simulink library "Feeder3_lib"  (Simulink 8.1)
settings: Solver=ode45  StartTime=0.0  StopTime=10.0  RelTol=1e-3
undefined symbols (not defined in the file): cable_spec, cb_mech_delay, Left, Ts, type, V
libraries: breaker_lib x11, transformer_lib x5, cables_lib x5, Load_lib x5, ssn_lib x3, rtlab x2, artemis x2
settings Model: Creator=re25624  LastModifiedBy=re25624

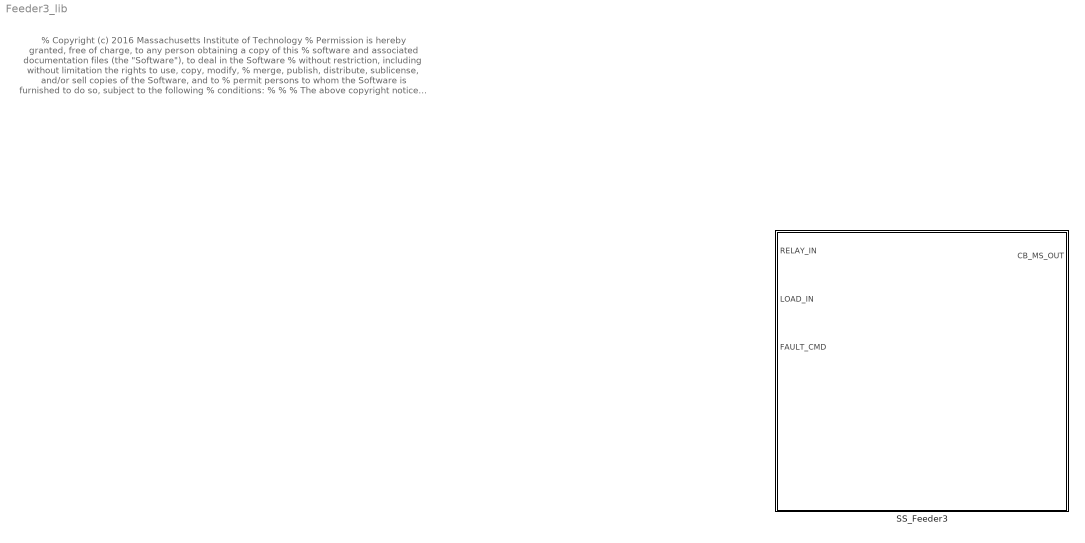
== system Feeder3_lib ==
  note: % Copyright (c) 2016 Massachusetts Institute of Technology
      | % Permission is hereby granted, free of charge, to any person obtaining a copy of this
      | % software and associated documentation files (the "Software"), to deal in the Software
      | % without restriction, including without limitation the rights to use, copy, modify,
      | % merge, publish, distribute, sublicense, and/or sell copies of the Software, and to
      | % permit persons to whom the Software is furnished to do so, subject to the following
      | % conditions:
      | %
      | %
      | % The above copyright notice and this permission notice shall be included in
      | % all copies or substantial portions of the Software.
      | %
      | % THE SOFTWARE IS PROVIDED "AS IS", WITHOUT WARRANTY OF ANY KIND, EXPRESS OR IMPLIED,
      | % INCLUDING BUT NOT LIMITED TO THE WARRANTIES OF MERCHANTABILITY, FITNESS FOR A
      | % PARTICULAR PURPOSE AND NONINFRINGEMENT. IN NO EVENT SHALL THE AUTHORS OR COPYRIGHT
      | % HOLDERS BE LIABLE FOR ANY CLAIM, DAMAGES OR OTHER LIABILITY, WHETHER IN AN ACTION
      | % OF CONTRACT, TORT OR OTHERWISE, ARISING FROM, OUT OF OR IN CONNECTION WITH THE
      | % SOFTWARE OR THE USE OR OTHER DEALINGS IN THE SOFTWARE.
      | %
      | %
      | %%
  SS_Feeder3 : Subsystem

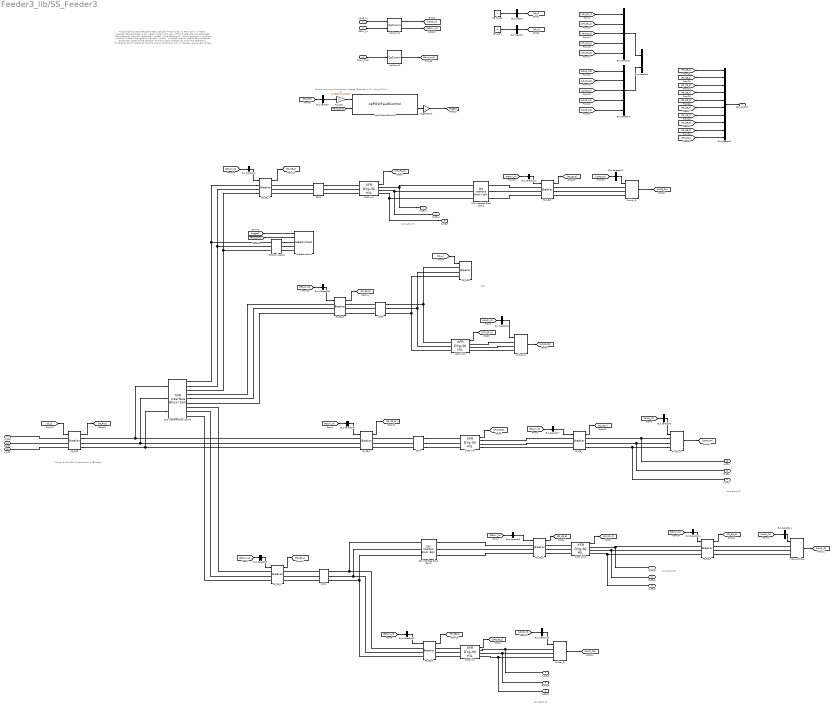
== system Feeder3_lib/SS_Feeder3 ==
  note: Point-on-wave synchronisation voltage (3-phase) in PU - Using 13.8 kV
  note: % Copyright (c) 2016 Massachusetts Institute of Technology
      | % Permission is hereby granted, free of charge, to any person obtaining a copy of this
      | % software and associated documentation files (the "Software"), to deal in the Software
      | % without restriction, including without limitation the rights to use, copy, modify,
      | % merge, publish, distribute, sublicense, and/or sell copies of the Software, and to
      | % permit persons to whom the Software is furnished to do so, subject to the following
      | % conditions:
      | %
      | %
      | % The above copyright notice and this permission notice shall be included in
      | % all copies or substantial portions of the Software.
      | %
      | % THE SOFTWARE IS PROVIDED "AS IS", WITHOUT WARRANTY OF ANY KIND, EXPRESS OR IMPLIED,
      | % INCLUDING BUT NOT LIMITED TO THE WARRANTIES OF MERCHANTABILITY, FITNESS FOR A
      | % PARTICULAR PURPOSE AND NONINFRINGEMENT. IN NO EVENT SHALL THE AUTHORS OR COPYRIGHT
      | % HOLDERS BE LIABLE FOR ANY CLAIM, DAMAGES OR OTHER LIABILITY, WHETHER IN AN ACTION
      | % OF CONTRACT, TORT OR OTHERWISE, ARISING FROM, OUT OF OR IN CONNECTION WITH THE
      | % SOFTWARE OR THE USE OR OTHER DEALINGS IN THE SOFTWARE.
      | %
      | %
      | %%
  note: connect to F1
  note: connect to F2
  note: connect to F2
  note: connect to F2
  note: CHP
  note: Signal for this Cb will come from a SEL relay
  RELAY_IN : Inport
  LOAD_IN : Inport  Port=2
  FAULT_CMD : Inport  Port=3
  1000 kVA : transformer_lib/XFR DYg-30 HIL  Rating=1000  Vp=13800  Vs=480  Z=5.56  XR=5.49
  1000 kVA1 : transformer_lib/XFR DYg-30 HIL  Rating=1000  Vp=13800  Vs=480  Z=5.56  XR=5.49
  2000 kVA : transformer_lib/XFR DYg-30 HIL  Rating=2000  Vp=13800  Vs=480  Z=5.75  XR=5.7
  2000 kVA1 : transformer_lib/XFR DYg-30 HIL  Rating=2000  Vp=13800  Vs=480  Z=5.75  XR=5.7
  2500 kVA : transformer_lib/XFR DYg-30 HIL  Rating=2500  Vp=13800  Vs=480  Z=5.75  XR=6.6
  500kcmil_cable : cables_lib/500kcmil_cable  length=1  par_sets=1
  Bus Creator : BusCreator  Inputs=1
  Bus Creator1 : BusCreator  Inputs=1
  Bus Creator2 : BusCreator  Inputs=5
  Bus Creator3 : BusCreator  Inputs=5
  Bus Creator4 : BusCreator  Inputs=2
  Bus Creator5 : BusCreator  Inputs=10
  Bus Selector : BusSelector  OutputSignals=Vabc_bus
  Bus Selector1 : BusSelector  OutputSignals=F3_CB_4
  Bus Selector10 : BusSelector  OutputSignals=F3_CB_5
  Bus Selector11 : BusSelector  OutputSignals=P6
  Bus Selector12 : BusSelector  OutputSignals=F3_CB_9
  Bus Selector13 : BusSelector  OutputSignals=F3_CB_3
  Bus Selector14 : BusSelector  OutputSignals=F3_CB_8
  Bus Selector2 : BusSelector  OutputSignals=C6
  Bus Selector3 : BusSelector  OutputSignals=P4
  Bus Selector4 : BusSelector  OutputSignals=I6
  Bus Selector5 : BusSelector  OutputSignals=C5
  Bus Selector6 : BusSelector  OutputSignals=F3_CB_2
  Bus Selector7 : BusSelector  OutputSignals=F3_CB_7
  Bus Selector8 : BusSelector  OutputSignals=F3_CB_6
  Bus Selector9 : BusSelector  OutputSignals=F3_CB_1
  C301 : cables_lib/PI-Section  cable_spec=[cable_spec(13, :)]  line_length=2500  parallel_sets=1
  C302 : cables_lib/PI-Section  cable_spec=[cable_spec(11, :)]  line_length=2000  parallel_sets=1
  C303 : cables_lib/PI-Section  cable_spec=[cable_spec(13, :)]  line_length=2000  parallel_sets=1
  C304 : cables_lib/PI-Section  cable_spec=[cable_spec(11, :)]  line_length=1500  parallel_sets=2
  CB closed : Constant
  CB open : Constant  Value=0
  Critical_5 : Load_lib/Dynamic_Load  V=460  Ts=Ts
  Critical_6 : Load_lib/Dynamic_Load  V=460  Ts=Ts
  F3_CB_{1..9} (9 alike) : breaker_lib/Breaker  Ts=Ts  mech_delays=[cb_mech_delay(1,:)]
  F3_GCB : breaker_lib/Breaker  Ts=Ts  mech_delays=[cb_mech_delay(1,:)]
  F3_PCC : breaker_lib/Breaker  Ts=Ts  mech_delays=[cb_mech_delay(1,:)]
  Interruptible_6 : Load_lib/Dynamic_Load  V=460  Ts=Ts
  OpComm1 : rtlab/OpComm  nbport=2  groupe_acq=1  subsys_rate=0  st=0  Synchronization=on  Interpolation=on  Threshold=1.0  Missed_Data=off  Sim_Time=off  Samples=off  dynSigOut=off  from_console=0  warning_done=off  writeOpCommFile=off  Offset=off
  OpComm2 : rtlab/OpComm  nbport=1  groupe_acq=1  subsys_rate=0  st=0  Synchronization=on  Interpolation=on  Threshold=1.0  Missed_Data=off  Sim_Time=off  Samples=off  dynSigOut=off  from_console=1  warning_done=off  writeOpCommFile=off  Offset=off
  Priority_4 : Load_lib/Dynamic_Load  V=460  Ts=Ts
  Priority_6 : Load_lib/Dynamic_Load  V=460  Ts=Ts
  SSN Interface Block (3ph)1 : ssn_lib/SSN Interface Block (3ph)  nb_phase=3  nb_port=2  p1_type=V-type(Left)  p2_type=V-type (Right)  p3_type=V-type(Left)  p4_type=V-type(Left)  p5_type=V-type(Left)  p6_type=V-type(Left)  p7_type=V-type(Left)  p8_type=V-type(Left)  p9_type=V-type(Left)  p10_type=V-type(Left)  p11_type=V-type(Left)  p12_type=V-type(Left)  p13_type=V-type(Left)  p14_type=V-type(Left)  p15_type=V-type(Left)  p16_type=V-type(Left)  I_port_shunt_resistance=1e9
  SSN Interface Block (3ph)2 : ssn_lib/SSN Interface Block (3ph)  nb_phase=3  nb_port=2  p1_type=V-type(Left)  p2_type=V-type (Right)  p3_type=V-type(Left)  p4_type=V-type(Left)  p5_type=V-type(Left)  p6_type=V-type(Left)  p7_type=V-type(Left)  p8_type=V-type(Left)  p9_type=V-type(Left)  p10_type=V-type(Left)  p11_type=V-type(Left)  p12_type=V-type(Left)  p13_type=V-type(Left)  p14_type=V-type(Left)  p15_type=V-type(Left)  p16_type=V-type(Left)  I_port_shunt_resistance=1e9
  SSN Interface Block (3ph)5 : ssn_lib/SSN Interface Block (3ph)  nb_phase=3  nb_port=4  p1_type=V-type(Left)  p2_type=V-type (Right)  p3_type=V-type (Right)  p4_type=V-type (Right)  p5_type=V-type(Left)  p6_type=V-type(Left)  p7_type=V-type(Left)  p8_type=V-type(Left)  p9_type=V-type(Left)  p10_type=V-type(Left)  p11_type=V-type(Left)  p12_type=V-type(Left)  p13_type=V-type(Left)  p14_type=V-type(Left)  p15_type=V-type(Left)  p16_type=V-type(Left)  I_port_shunt_resistance=1e9
  a : Gain  Gain=1/(13800*sqrt(2/3))
  opElectricFault : artemis/Tools /POW faults/opElectricFault  FaultLocation=location 4  FaultResistance=0.0001  GroundResistance=0.0001  InitialStates=[0 0 0]  SnubberResistance=1e6  SnubberCapacitance=inf
  opPOWFaultControl1 : artemis/Tools /POW faults/opPOWFaultControl  Ts=Ts  usePLL=off  Fgrid=60  PLL_k=[180 3200 1]  vol_sel=1: rising zero-corssing  SyncPhase_menu=A  T_acq=0.8
  triggerFAULT : Gain
  A_CB_4 : PMIOPort  Port=1  Side=Right
  B_CB_4 : PMIOPort  Port=2  Side=Right
  C_CB_4 : PMIOPort  Port=3  Side=Right
  A_CB_5 : PMIOPort  Port=4  Side=Right
  B_CB_5 : PMIOPort  Port=5  Side=Right
  C_CB_5 : PMIOPort  Port=6  Side=Right
  A_CB_6 : PMIOPort  Port=7  Side=Right
  B_CB_6 : PMIOPort  Port=8  Side=Right
  C_CB_6 : PMIOPort  Port=9  Side=Right
  A_CB_7 : PMIOPort  Port=10  Side=Right
  B_CB_7 : PMIOPort  Port=11  Side=Right
  C_CB_7 : PMIOPort  Port=12  Side=Right
  A_PCC : PMIOPort  Port=13  Side=Left
  B_PCC : PMIOPort  Port=14  Side=Left
  C_PCC : PMIOPort  Port=15  Side=Left
  CB_MS_OUT : Outport
  wires:
  FAULT_CMD/1 -> OpComm2/1
  OpComm2/1 -> [fault_cmd]
  [trigger] -> opElectricFault/1
  [fault_cmd] -> opElectricFault/2
  a/1 -> opPOWFaultControl1/1
  Bus Selector/1 -> a/1  "<Vabc_bus>"
  [F3_PCC] -> Bus Selector/1
  triggerFAULT/1 -> [trigger]  "triggerFAULTsig"
  opPOWFaultControl1/2 -> triggerFAULT/1
  [fault_cmd] -> opPOWFaultControl1/2
  [F3_CB_9] -> Bus Creator5/9  "F3_CB_9"
  [F3_CB_8] -> Bus Creator5/8  "F3_CB_8"
  [RELAY_IN] -> Bus Selector14/1
  Bus Selector14/1 -> F3_CB_8/1  "<F3_CB_8>"
  F3_CB_8/1 -> [F3_CB_8]
  [RELAY_IN] -> Bus Selector12/1
  Bus Selector12/1 -> F3_CB_9/1  "<F3_CB_9>"
  F3_CB_9/1 -> [F3_CB_9]
  [LOAD_P6] -> Bus Creator3/5  "F3_P6"
  Priority_6/1 -> [LOAD_P6]
  Bus Selector11/1 -> Priority_6/1  "<P6>"
  [LOAD_IN] -> Bus Selector11/1
  [F3_PCC] -> Bus Creator5/10  "F3_PCC"
  F3_PCC/1 -> [F3_PCC]
  F3_CB_7/1 -> [F3_CB_7]
  2500 kVA/1 -> [XFM_F3_5]
  [cb_o] -> F3_GCB/1
  [cb_c] -> F3_PCC/1
  [RELAY_IN] -> Bus Selector13/1
  Bus Selector13/1 -> F3_CB_3/1  "<F3_CB_3>"
  [RELAY_IN] -> Bus Selector10/1
  Bus Selector10/1 -> F3_CB_5/1  "<F3_CB_5>"
  [RELAY_IN] -> Bus Selector9/1
  Bus Selector9/1 -> F3_CB_1/1  "<F3_CB_1>"
  [RELAY_IN] -> Bus Selector8/1
  Bus Selector8/1 -> F3_CB_6/1  "<F3_CB_6>"
  [RELAY_IN] -> Bus Selector7/1
  Bus Selector7/1 -> F3_CB_7/1  "<F3_CB_7>"
  [RELAY_IN] -> Bus Selector6/1
  Bus Selector6/1 -> F3_CB_2/1  "<F3_CB_2>"
  OpComm1/2 -> [RELAY_IN]
  RELAY_IN/1 -> OpComm1/2
  [RELAY_IN] -> Bus Selector1/1
  Bus Creator5/1 -> CB_MS_OUT/1
  [F3_CB_4] -> Bus Creator5/4  "F3_CB_4"
  [F3_CB_2] -> Bus Creator5/2  "F3_CB_2"
  [F3_CB_3] -> Bus Creator5/3  "F3_CB_3"
  [F3_CB_6] -> Bus Creator5/6  "F3_CB_6"
  [F3_CB_7] -> Bus Creator5/7  "F3_CB_7"
  [F3_CB_5] -> Bus Creator5/5  "F3_CB_5"
  [F3_CB_1] -> Bus Creator5/1  "F3_CB_1"
  F3_CB_5/1 -> [F3_CB_5]
  F3_CB_1/1 -> [F3_CB_1]
  F3_CB_6/1 -> [F3_CB_6]
  F3_CB_2/1 -> [F3_CB_2]
  F3_CB_3/1 -> [F3_CB_3]
  F3_CB_4/1 -> [F3_CB_4]
  Bus Creator3/1 -> Bus Creator4/2  "LOAD"
  Bus Creator2/1 -> Bus Creator4/1  "XFR"
  [LOAD_P4] -> Bus Creator3/4  "F3_P4"
  [LOAD_I6] -> Bus Creator3/3  "F3_I6"
  [LOAD_C5] -> Bus Creator3/1  "F3_C5"
  [LOAD_C6] -> Bus Creator3/2  "F3_C6"
  Critical_5/1 -> [LOAD_C5]
  Interruptible_6/1 -> [LOAD_I6]
  Priority_4/1 -> [LOAD_P4]
  Critical_6/1 -> [LOAD_C6]
  [XFM_F3_4] -> Bus Creator2/4  "F3_X4"
  [XFM_F3_3] -> Bus Creator2/3  "F3_X3"
  [XFM_F3_5] -> Bus Creator2/5  "F3_X5"
  [XFM_F3_1] -> Bus Creator2/1  "F3_X1"
  [XFM_F3_2] -> Bus Creator2/2  "F3_X2"
  1000 kVA1/1 -> [XFM_F3_4]
  1000 kVA/1 -> [XFM_F3_3]
  2000 kVA1/1 -> [XFM_F3_2]
  2000 kVA/1 -> [XFM_F3_1]
  Bus Selector5/1 -> Critical_5/1  "<C5>"
  Bus Selector4/1 -> Interruptible_6/1  "<I6>"
  Bus Selector3/1 -> Priority_4/1  "<P4>"
  Bus Selector2/1 -> Critical_6/1  "<C6>"
  [LOAD_IN] -> Bus Selector5/1
  [LOAD_IN] -> Bus Selector4/1
  [LOAD_IN] -> Bus Selector3/1
  [LOAD_IN] -> Bus Selector2/1
  OpComm1/1 -> [LOAD_IN]
  LOAD_IN/1 -> OpComm1/1
  CB open/1 -> Bus Creator1/1  "Logic_trip"
  Bus Selector1/1 -> F3_CB_4/1  "<F3_CB_4>"
  Bus Creator1/1 -> [cb_o]
  Bus Creator/1 -> [cb_c]
  CB closed/1 -> Bus Creator/1  "Logic_trip"
  connections:
  SSN Interface Block (3ph)2/RConn1 -- F3_CB_9/LConn1
  SSN Interface Block (3ph)2/RConn3 -- F3_CB_9/LConn3
  SSN Interface Block (3ph)2/RConn2 -- F3_CB_9/LConn2
  500kcmil_cable/RConn1 -- opElectricFault/LConn1
  500kcmil_cable/RConn3 -- opElectricFault/LConn3
  500kcmil_cable/RConn2 -- opElectricFault/LConn2
  SSN Interface Block (3ph)5/LConn2 -- F3_CB_2/LConn2 -- F3_PCC/RConn2
  SSN Interface Block (3ph)5/LConn3 -- F3_CB_2/LConn3 -- F3_PCC/RConn3
  SSN Interface Block (3ph)5/LConn1 -- F3_CB_2/LConn1 -- F3_PCC/RConn1
  F3_PCC/LConn1 -- A_PCC/RConn1
  F3_PCC/LConn3 -- C_PCC/RConn1
  F3_PCC/LConn2 -- B_PCC/RConn1
  C303/RConn1 -- 2500 kVA/LConn1
  C303/RConn3 -- 2500 kVA/LConn3
  C303/RConn2 -- 2500 kVA/LConn2
  C303/LConn3 -- F3_CB_4/RConn3
  C303/LConn2 -- F3_CB_4/RConn2
  C303/LConn1 -- F3_CB_4/RConn1
  SSN Interface Block (3ph)1/RConn3 -- F3_CB_6/LConn3
  SSN Interface Block (3ph)1/RConn1 -- F3_CB_6/LConn1
  SSN Interface Block (3ph)1/RConn2 -- F3_CB_6/LConn2
  F3_CB_1/LConn3 -- SSN Interface Block (3ph)5/RConn9
  F3_CB_1/LConn2 -- SSN Interface Block (3ph)5/RConn8
  F3_CB_1/LConn1 -- SSN Interface Block (3ph)5/RConn7
  SSN Interface Block (3ph)5/RConn5 -- F3_CB_3/LConn2
  SSN Interface Block (3ph)5/RConn6 -- F3_CB_3/LConn3
  SSN Interface Block (3ph)5/RConn4 -- F3_CB_3/LConn1
  F3_CB_4/LConn2 -- 500kcmil_cable/LConn2 -- SSN Interface Block (3ph)5/RConn2
  F3_CB_4/LConn3 -- 500kcmil_cable/LConn3 -- SSN Interface Block (3ph)5/RConn3
  F3_CB_4/LConn1 -- 500kcmil_cable/LConn1 -- SSN Interface Block (3ph)5/RConn1
  F3_CB_8/RConn3 -- Interruptible_6/LConn3
  F3_CB_8/RConn2 -- Interruptible_6/LConn2
  F3_CB_8/RConn1 -- Interruptible_6/LConn1
  F3_CB_9/RConn3 -- Priority_6/LConn3
  F3_CB_9/RConn2 -- Priority_6/LConn2
  F3_CB_9/RConn1 -- Priority_6/LConn1
  1000 kVA/RConn1 -- F3_CB_7/LConn1
  1000 kVA/RConn2 -- F3_CB_7/LConn2
  1000 kVA/RConn3 -- F3_CB_7/LConn3
  C304/RConn1 -- 1000 kVA/LConn1
  C304/RConn3 -- 1000 kVA/LConn3
  C304/RConn2 -- 1000 kVA/LConn2
  B_CB_4/RConn1 -- SSN Interface Block (3ph)2/LConn2 -- 2500 kVA/RConn2
  C_CB_4/RConn1 -- SSN Interface Block (3ph)2/LConn3 -- 2500 kVA/RConn3
  A_CB_4/RConn1 -- SSN Interface Block (3ph)2/LConn1 -- 2500 kVA/RConn1
  Critical_5/LConn2 -- B_CB_5/RConn1 -- 2000 kVA/RConn2
  Critical_5/LConn3 -- C_CB_5/RConn1 -- 2000 kVA/RConn3
  2000 kVA/RConn1 -- A_CB_5/RConn1 -- Critical_5/LConn1
  2000 kVA1/RConn2 -- B_CB_6/RConn1 -- F3_CB_8/LConn2
  F3_CB_8/LConn3 -- C_CB_6/RConn1 -- 2000 kVA1/RConn3
  2000 kVA1/RConn1 -- A_CB_6/RConn1 -- F3_CB_8/LConn1
  Priority_4/LConn2 -- B_CB_7/RConn1 -- F3_CB_7/RConn2
  Priority_4/LConn3 -- C_CB_7/RConn1 -- F3_CB_7/RConn3
  Priority_4/LConn1 -- A_CB_7/RConn1 -- F3_CB_7/RConn1
  C304/LConn3 -- F3_CB_2/RConn3
  F3_CB_5/RConn3 -- 2000 kVA/LConn3
  F3_CB_5/RConn1 -- 2000 kVA/LConn1
  C302/LConn1 -- F3_CB_3/RConn1
  F3_CB_6/RConn1 -- 2000 kVA1/LConn1
  C304/LConn2 -- F3_CB_2/RConn2
  SSN Interface Block (3ph)1/LConn2 -- C301/RConn2 -- F3_CB_5/LConn2
  C302/LConn3 -- F3_CB_3/RConn3
  F3_CB_5/RConn2 -- 2000 kVA/LConn2
  C301/LConn1 -- F3_CB_1/RConn1
  F3_GCB/LConn2 -- C302/RConn2 -- 1000 kVA1/LConn2
  F3_CB_6/RConn2 -- 2000 kVA1/LConn2
  F3_GCB/LConn1 -- C302/RConn1 -- 1000 kVA1/LConn1
  C302/LConn2 -- F3_CB_3/RConn2
  F3_GCB/LConn3 -- C302/RConn3 -- 1000 kVA1/LConn3
  C304/LConn1 -- F3_CB_2/RConn1
  C301/LConn3 -- F3_CB_1/RConn3
  Critical_6/LConn3 -- 1000 kVA1/RConn3
  SSN Interface Block (3ph)1/LConn3 -- C301/RConn3 -- F3_CB_5/LConn3
  Critical_6/LConn1 -- 1000 kVA1/RConn1
  C301/LConn2 -- F3_CB_1/RConn2
  Critical_6/LConn2 -- 1000 kVA1/RConn2
  F3_CB_6/RConn3 -- 2000 kVA1/LConn3
  SSN Interface Block (3ph)1/LConn1 -- C301/RConn1 -- F3_CB_5/LConn1
